simulink model "test_sf_tm_turb"  (R2013b)
settings: Solver=FixedStepDiscrete  StartTime=0.0  StopTime=1  FixedStep=1/1200  RelTol=1e-3
settings Model: Creator=HSidaoui  LastModifiedBy=AGSilva
settings OptimizationCC: ExpressionDepthLimit=2147483647
settings DebuggingCC: StateNameClashWarn=warning

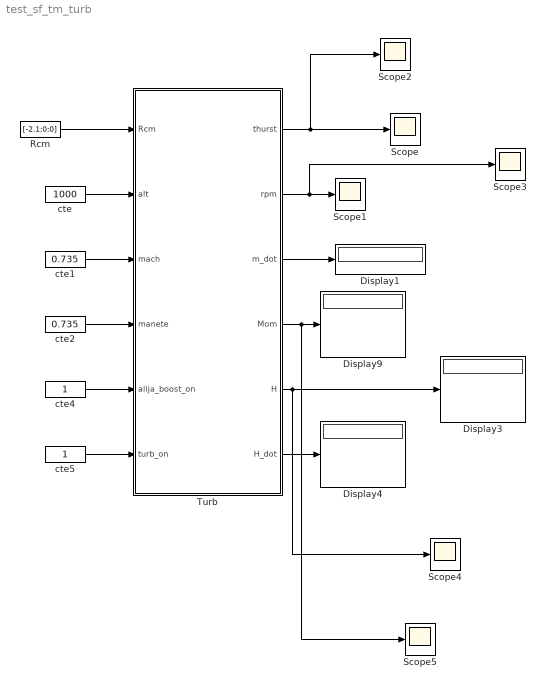
== system test_sf_tm_turb ==
  Display{1,3..4,9} (4 alike) : Display
  Rcm : Constant  Value=[-2.1;0;0]
  Scope{,1..5} (6 alike) : Scope
      Scope2 settings: SaveName=ScopeData2
      Scope3 settings: SaveName=ScopeData3
      Scope4 settings: SaveName=ScopeData4
      Scope5 settings: SaveName=ScopeData5
  Turb : Subsystem  TreatAsAtomicUnit=on
  cte : Constant  Value=1000
  cte1 : Constant  Value=0.735
  cte2 : Constant  Value=0.735
  cte4 : Constant
  cte5 : Constant
  wires:
  cte/1 -> Turb/2(alt)
  Turb/3(m_dot) -> Display1/1
  cte1/1 -> Turb/3(mach)
  Turb/4(Mom) -> Scope5/1, Display9/1
  Rcm/1 -> Turb/1(Rcm)
  cte2/1 -> Turb/4(manete)
  cte5/1 -> Turb/6(turb_on)
  cte4/1 -> Turb/5(alija_boost_on)
  Turb/5(H) -> Scope4/1, Display3/1
  Turb/6(H_dot) -> Display4/1
  Turb/1(thurst) -> Scope2/1, Scope/1
  Turb/2(rpm) -> Scope3/1, Scope1/1

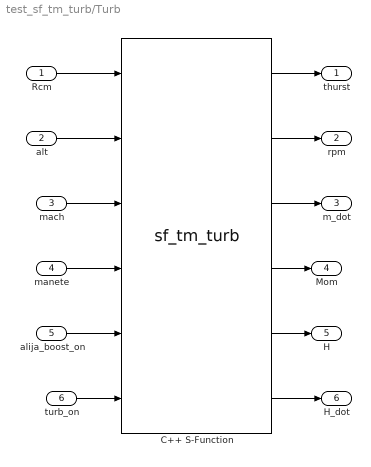
== system test_sf_tm_turb/Turb ==
  Rcm : Inport
  alt : Inport  Port=2
  mach : Inport  Port=3
  manete : Inport  Port=4
  alija_boost_on : Inport  Port=5
  turb_on : Inport  Port=6
  C++ S-Function : S-Function  FunctionName=sf_tm_turb  EnableBusSupport=off
  thurst : Outport
  rpm : Outport  Port=2
  m_dot : Outport  Port=3
  Mom : Outport  Port=4
  H : Outport  Port=5
  H_dot : Outport  Port=6
  wires:
  Rcm/1 -> C++ S-Function/1
  alt/1 -> C++ S-Function/2
  mach/1 -> C++ S-Function/3
  manete/1 -> C++ S-Function/4
  alija_boost_on/1 -> C++ S-Function/5
  turb_on/1 -> C++ S-Function/6
  C++ S-Function/6 -> H_dot/1
  C++ S-Function/5 -> H/1
  C++ S-Function/1 -> thurst/1
  C++ S-Function/2 -> rpm/1
  C++ S-Function/3 -> m_dot/1
  C++ S-Function/4 -> Mom/1
